simulink model "my_simulation_model"  (R2024b)
settings: Solver=VariableStepAuto  StartTime=0.0  StopTime=10.0  RelTol=1e-3
settings Model: Creator=xinxing  LastModifiedBy=xinxing

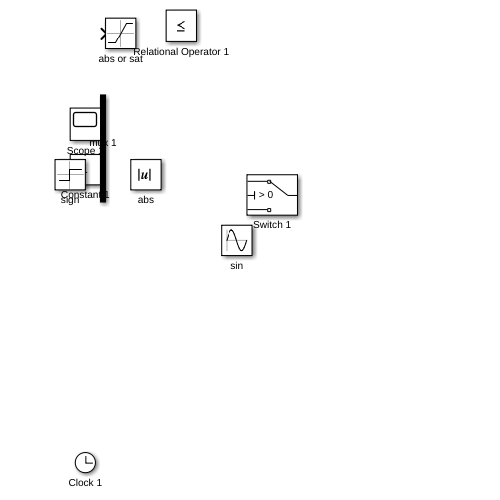
[thumbnail: Simulink's stored preview of the top-level diagram]
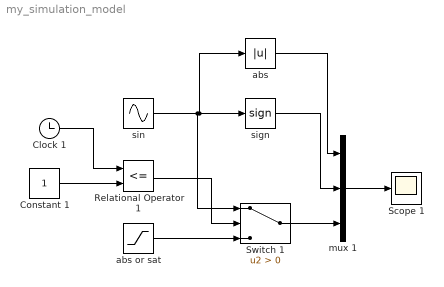
== system my_simulation_model ==
  Clock 1 : Clock
  Constant 1 : Constant
  Relational Operator 1 : RelationalOperator  Operator=<=  OutDataTypeStr=boolean  RndMeth=Simplest  InputSameDT=off
  Scope 1 : Scope
  Switch 1 : Switch  Criteria=u2 > Threshold  SaturateOnIntegerOverflow=off  InputSameDT=off
  abs : Abs  SaturateOnIntegerOverflow=off
  abs or sat : Saturate
  mux 1 : Mux  Inputs=3
  sign : Signum
  sin : Sin  SampleTime=0
  wires:
  Switch 1/1 -> mux 1/3
  sign/1 -> mux 1/2
  abs/1 -> mux 1/1
  Relational Operator 1/1 -> Switch 1/2
  sin/1 -> sign/1, abs/1, Switch 1/1
  mux 1/1 -> Scope 1/1
  Constant 1/1 -> Relational Operator 1/2
  abs or sat/1 -> Switch 1/3
  Clock 1/1 -> Relational Operator 1/1
